simulink model "Problem2Group10"  (R2023b)
settings: Solver=VariableStepAuto  StartTime=0.0  StopTime=10.0  RelTol=1e-3
values from neighbouring files (symbols this model uses):
  G1_den = [1 0 0]    [Lab3_Number1Codes.m]    (also in Problem2Group10.m)
  G1_num = [0 0 1]    [Lab3_Number1Codes.m]    (also in Problem2Group10.m = [1])
  G2_den = [1 1]    [Lab3_Number1Codes.m]    (also in Problem2Group10.m)
  G2_num = [0 1]    [Lab3_Number1Codes.m]    (also in Problem2Group10.m = [1])
  G3_den = [1 0]    [Lab3_Number1Codes.m]    (also in Problem2Group10.m)
  G3_num = [0 1]    [Lab3_Number1Codes.m]    (also in Problem2Group10.m = [1])
  G4_den = [2 0]    [Problem2Group10.m]
  G4_num = [1]    [Problem2Group10.m]
  H1_den = [1 0]    [Lab3_Number1Codes.m]    (also in Problem2Group10.m)
  H1_num = [0 1]    [Lab3_Number1Codes.m]    (also in Problem2Group10.m = [1])
  H2_den = [1 -1]    [Lab3_Number1Codes.m]    (also in Problem2Group10.m)
  H2_num = [0 1]    [Lab3_Number1Codes.m]    (also in Problem2Group10.m = [1])
  H3_den = [1 -2]    [Lab3_Number1Codes.m]    (also in Problem2Group10.m)
  H3_num = [0 1]    [Lab3_Number1Codes.m]    (also in Problem2Group10.m = [1])
  TF3_den = conv(G3_den,TF3_add)    [Lab3_Number1Codes.m]    (also in Problem2Group10.m = conv(G1G4TF2_den_H1_den_G1G4TF2_num_H1_num_sum, G1G4TF2_den))
  TF3_num = conv(GH3_den,GH3_num)    [Lab3_Number1Codes.m]    (also in Problem2Group10.m = conv(G1G4TF2_num_G1G4TF2_den, H1_den))
settings Model: Creator=Poopy  LastModifiedBy=Acer

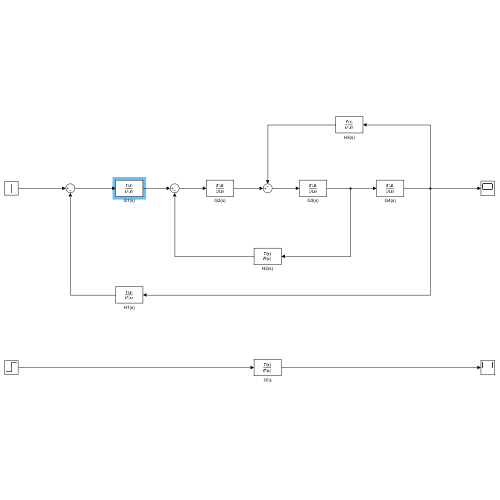
[thumbnail: Simulink's stored preview of the top-level diagram]
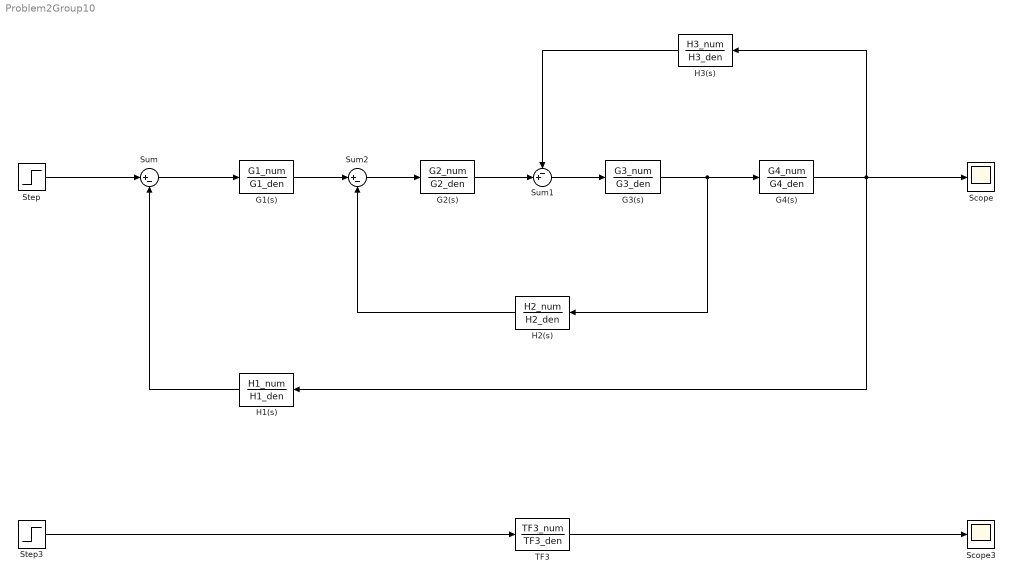
== system Problem2Group10 ==
  G1(s) : TransferFcn  Numerator=G1_num  Denominator=G1_den
  G2(s) : TransferFcn  Numerator=G2_num  Denominator=G2_den
  G3(s) : TransferFcn  Numerator=G3_num  Denominator=G3_den
  G4(s) : TransferFcn  Numerator=G4_num  Denominator=G4_den
  H1(s) : TransferFcn  Numerator=H1_num  Denominator=H1_den
  H2(s) : TransferFcn  Numerator=H2_num  Denominator=H2_den
  H3(s) : TransferFcn  Numerator=H3_num  Denominator=H3_den
  Scope : Scope
  Scope3 : Scope
  Step : Step  Time=0  SampleTime=0
  Step3 : Step  Time=0  SampleTime=0
  Sum : Sum  Inputs=|+-
  Sum1 : Sum  Inputs=-+|
  Sum2 : Sum  Inputs=|+-
  TF3 : TransferFcn  Numerator=TF3_num  Denominator=TF3_den
  wires:
  G1(s)/1 -> Sum2/1
  H2(s)/1 -> Sum2/2
  G4(s)/1 -> H1(s)/1, Scope/1, H3(s)/1
  G3(s)/1 -> H2(s)/1, G4(s)/1
  Step3/1 -> TF3/1
  G2(s)/1 -> Sum1/2
  Sum/1 -> G1(s)/1
  H3(s)/1 -> Sum1/1
  Sum2/1 -> G2(s)/1
  Step/1 -> Sum/1
  H1(s)/1 -> Sum/2
  TF3/1 -> Scope3/1
  Sum1/1 -> G3(s)/1
